simulink library "calcAeroCoeffFromPolynomial_ul"  (R2020a)
settings: Solver=VariableStepAuto  StartTime=0.0  StopTime=10.0  RelTol=1e-3
undefined symbols (not defined in the file): coeffvals
libraries: dsppolyfun x1
settings Model: Creator=Ayaz  LastModifiedBy=Ayaz

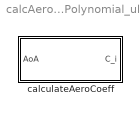
== system calcAeroCoeffFromPolynomial_ul ==
  calculateAeroCoeff : Subsystem  mask{coeffVals=coeffvals}
      mask prompts: coeffVals "Polynomial coefficient values: (c0,c1,c2)"
      mask TypeOptions coeffVals: coeffvals/Value

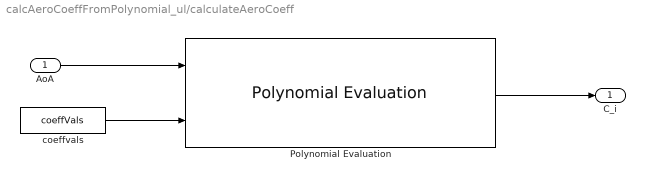
== system calcAeroCoeffFromPolynomial_ul/calculateAeroCoeff ==
  AoA : Inport
  Polynomial Evaluation : dsppolyfun/Polynomial Evaluation  useConstCoeffs=off  constCoeffs=[5 4 3 2 1]
      settings: SourceProductBaseCode=DS
  coeffvals : Constant  Value=coeffVals
  C_i : Outport
  wires:
  coeffvals/1 -> Polynomial Evaluation/2
  AoA/1 -> Polynomial Evaluation/1
  Polynomial Evaluation/1 -> C_i/1
